simulink model "myMat2"  (R2020b)
settings: Solver=VariableStepAuto  StartTime=0.0  StopTime=200  RelTol=1e-3
libraries: pid_lib x2, simulink x2
settings Model: Creator=jsoudier01  LastModifiedBy=xoxox
settings DataIOCC: ReturnWorkspaceOutputs=off
settings DebuggingCC: ArithmeticOperatorsInVariantConditions=warning
settings SFSimCC: SimUseLocalCustomCode=off  CustomCodeUndefinedFunction=UseInterfaceOnly
settings RTWCC: RTWUseLocalCustomCode=off

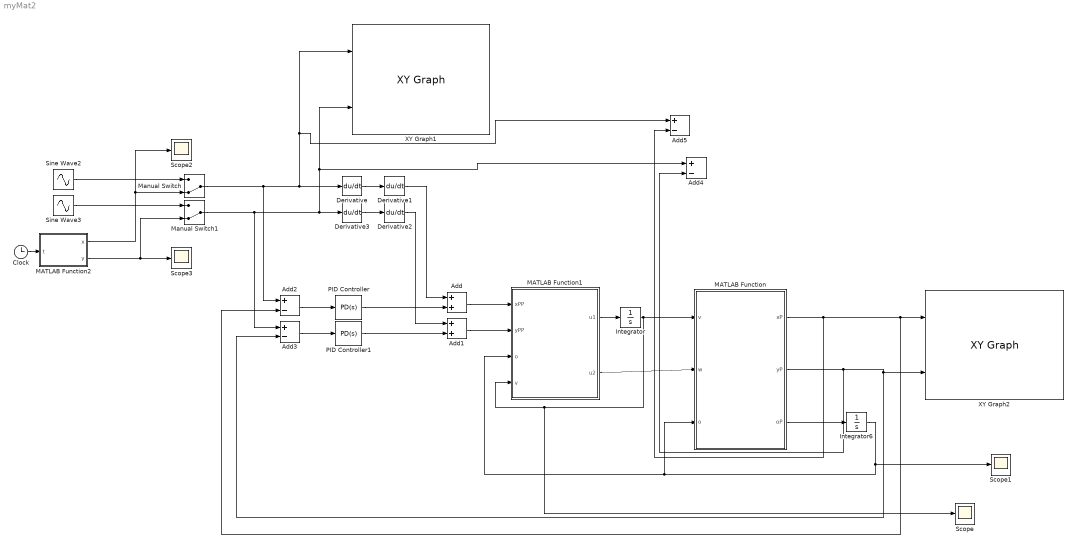
== system myMat2 ==
  Add : Sum
  Add1 : Sum
  Add{2..5} (4 alike) : Sum  Inputs=+-
  Clock : Clock
  Derivative{,1..3} (4 alike) : Derivative
  Integrator : Integrator  InitialCondition=50
  Integrator6 : Integrator  InitialCondition=10
  MATLAB Function : MATLAB Function  TreatAsAtomicUnit=on
  MATLAB Function1 : MATLAB Function  TreatAsAtomicUnit=on
  MATLAB Function2 : MATLAB Function  TreatAsAtomicUnit=on
  Manual Switch : ManualSwitch  CurrentSetting=0
  Manual Switch1 : ManualSwitch  CurrentSetting=0
  PID Controller : pid_lib/PID Controller  Controller=PD  Form=Ideal  TimeDomain=Continuous-time  UseExternalTs=off  SampleTime=-1  IntegratorMethod=Forward Euler  FilterMethod=Forward Euler  ControllerParametersSource=internal  P=1  I=1  D=1  UseFilter=on  N=100  TunerSelectOption=Transfer Function Based (PID Tuner App)  InitialConditionSource=internal  InitialConditionForIntegrator=0  InitialConditionForFilter=0  DifferentiatorICPrevScaledInput=0  ExternalReset=none  TrackingMode=off  Kt=1  LimitOutput=off  SatLimitsSource=internal  UpperSaturationLimit=inf  LowerSaturationLimit=-inf  LinearizeAsGain=on  AntiWindupMode=none  Kb=1  POutMin=[]  POutMax=[]  IOutMin=[]  IOutMax=[]  DOutMin=[]  DOutMax=[]  NOutMin=[]  NOutMax=[]  SumOutMin=[]  SumOutMax=[]  SaturationOutMin=[]  SaturationOutMax=[]  PParamMin=[]  PParamMax=[]  IParamMin=[]  IParamMax=[]  DParamMin=[]  DParamMax=[]  NParamMin=[]  NParamMax=[]  KbParamMin=[]  KbParamMax=[]  KtParamMin=[]  KtParamMax=[]  KbOutMin=[]  KbOutMax=[]  KtOutMin=[]  KtOutMax=[]  IntegratorOutMin=[]  IntegratorOutMax=[]  FilterOutMin=[]  FilterOutMax=[]  SumI1OutMin=[]  SumI1OutMax=[]  SumI2OutMin=[]  SumI2OutMax=[]  SumI3OutMin=[]  SumI3OutMax=[]  SumI4OutMin=[]  SumI4OutMax=[]  SumDOutMin=[]  SumDOutMax=[]  DifferentiatorOutMin=[]  DifferentiatorOutMax=[]  FilterDiffOutCoefMin=[]  FilterDiffOutCoefMax=[]  ReciprocalOutMin=[]  ReciprocalOutMax=[]  SumDenOutMin=[]  SumDenOutMax=[]  SumNumOutMin=[]  SumNumOutMax=[]  DivideOutMin=[]  DivideOutMax=[]  UdiffTsProdOutMin=[]  UdiffTsProdOutMax=[]  NTsProdOutMin=[]  NTsProdOutMax=[]  UintegralTsProdOutMin=[]  UintegralTsProdOutMax=[]  UngainTsProdOutMin=[]  UngainTsProdOutMax=[]  IntegratorContinuousStateAttributes=''  IntegratorStateMustResolveToSignalObject=off  IntegratorRTWStateStorageClass=Auto  FilterContinuousStateAttributes=''  FilterStateMustResolveToSignalObject=off  FilterRTWStateStorageClass=Auto  ParallelPVariant=Passthrough  IdealPVariant=InternalParameters  IVariant=Disabled  DVariant=InternalParameters  IntegratorVariant=Disabled  SatVariant=Disabled  AWVariant=Disabled  PCopyVariant=Disabled  TRVariant=Disabled  FdbkBlocksVariant=Forward  IdealPFdbkVariant=Disabled  SatFdbkVariant=Disabled  DerivativeFilterVariant=ContFilter  NVariant=InternalParameters  NCopyVariant=Disabled  FilterICVariant=InternalICsFilter  IntegratorICVariant=Disabled  ExternalResetVariant=Disabled  TRSumVariant=Passthrough  SumFdbkVariant=Disabled  SumVariant=Sum_PD  TsampFilterVariant=InternalTs  TsampNgainVariant=Passthrough  TsampIntegralVariant=Disabled_SignalSpec  ExternalSaturationOutDataTypeStr=Inherit: Same as second input
  PID Controller1 : pid_lib/PID Controller  Controller=PD  Form=Ideal  TimeDomain=Continuous-time  UseExternalTs=off  SampleTime=-1  IntegratorMethod=Forward Euler  FilterMethod=Forward Euler  ControllerParametersSource=internal  P=1  I=1  D=1  UseFilter=on  N=100  TunerSelectOption=Transfer Function Based (PID Tuner App)  InitialConditionSource=internal  InitialConditionForIntegrator=0  InitialConditionForFilter=0  DifferentiatorICPrevScaledInput=0  ExternalReset=none  TrackingMode=off  Kt=1  LimitOutput=off  SatLimitsSource=internal  UpperSaturationLimit=inf  LowerSaturationLimit=-inf  LinearizeAsGain=on  AntiWindupMode=none  Kb=1  POutMin=[]  POutMax=[]  IOutMin=[]  IOutMax=[]  DOutMin=[]  DOutMax=[]  NOutMin=[]  NOutMax=[]  SumOutMin=[]  SumOutMax=[]  SaturationOutMin=[]  SaturationOutMax=[]  PParamMin=[]  PParamMax=[]  IParamMin=[]  IParamMax=[]  DParamMin=[]  DParamMax=[]  NParamMin=[]  NParamMax=[]  KbParamMin=[]  KbParamMax=[]  KtParamMin=[]  KtParamMax=[]  KbOutMin=[]  KbOutMax=[]  KtOutMin=[]  KtOutMax=[]  IntegratorOutMin=[]  IntegratorOutMax=[]  FilterOutMin=[]  FilterOutMax=[]  SumI1OutMin=[]  SumI1OutMax=[]  SumI2OutMin=[]  SumI2OutMax=[]  SumI3OutMin=[]  SumI3OutMax=[]  SumI4OutMin=[]  SumI4OutMax=[]  SumDOutMin=[]  SumDOutMax=[]  DifferentiatorOutMin=[]  DifferentiatorOutMax=[]  FilterDiffOutCoefMin=[]  FilterDiffOutCoefMax=[]  ReciprocalOutMin=[]  ReciprocalOutMax=[]  SumDenOutMin=[]  SumDenOutMax=[]  SumNumOutMin=[]  SumNumOutMax=[]  DivideOutMin=[]  DivideOutMax=[]  UdiffTsProdOutMin=[]  UdiffTsProdOutMax=[]  NTsProdOutMin=[]  NTsProdOutMax=[]  UintegralTsProdOutMin=[]  UintegralTsProdOutMax=[]  UngainTsProdOutMin=[]  UngainTsProdOutMax=[]  IntegratorContinuousStateAttributes=''  IntegratorStateMustResolveToSignalObject=off  IntegratorRTWStateStorageClass=Auto  FilterContinuousStateAttributes=''  FilterStateMustResolveToSignalObject=off  FilterRTWStateStorageClass=Auto  ParallelPVariant=Passthrough  IdealPVariant=InternalParameters  IVariant=Disabled  DVariant=InternalParameters  IntegratorVariant=Disabled  SatVariant=Disabled  AWVariant=Disabled  PCopyVariant=Disabled  TRVariant=Disabled  FdbkBlocksVariant=Forward  IdealPFdbkVariant=Disabled  SatFdbkVariant=Disabled  DerivativeFilterVariant=ContFilter  NVariant=InternalParameters  NCopyVariant=Disabled  FilterICVariant=InternalICsFilter  IntegratorICVariant=Disabled  ExternalResetVariant=Disabled  TRSumVariant=Passthrough  SumFdbkVariant=Disabled  SumVariant=Sum_PD  TsampFilterVariant=InternalTs  TsampNgainVariant=Passthrough  TsampIntegralVariant=Disabled_SignalSpec  ExternalSaturationOutDataTypeStr=Inherit: Same as second input
  Scope{,1..3} (4 alike) : Scope
  Sine Wave2 : Sin  Frequency=1/10  SampleTime=0
  Sine Wave3 : Sin  Frequency=1/20  SampleTime=0
  XY Graph1 : simulink/Sinks/XY Graph  xmin=-10  xmax=10  ymin=-10  ymax=10  st=-1
  XY Graph2 : simulink/Sinks/XY Graph  xmin=-100  xmax=100  ymin=-100  ymax=100  st=-1
  wires:
  Manual Switch/1 -> Add2/1, Add5/1, XY Graph1/1, Derivative/1
  Derivative/1 -> Derivative1/1
  Manual Switch1/1 -> Add3/1, Add4/1, XY Graph1/2, Derivative3/1
  Derivative3/1 -> Derivative2/1
  MATLAB Function/3(oP) -> Integrator6/1
  Integrator6/1 -> Scope1/1, MATLAB Function1/3(o), MATLAB Function/3(o)
  MATLAB Function1/2(u2) -> MATLAB Function/2(w)
  MATLAB Function1/1(u1) -> Integrator/1
  Integrator/1 -> Scope/1, MATLAB Function1/4(v), MATLAB Function/1(v)
  MATLAB Function/1(xP) -> Add5/2, XY Graph2/1, Add2/2
  MATLAB Function/2(yP) -> Add4/2, XY Graph2/2, Add3/2
  Add/1 -> MATLAB Function1/1(xPP)
  Add1/1 -> MATLAB Function1/2(yPP)
  Derivative1/1 -> Add/1
  Derivative2/1 -> Add1/1
  Add3/1 -> PID Controller1/1
  Add2/1 -> PID Controller/1
  PID Controller/1 -> Add/2
  PID Controller1/1 -> Add1/2
  Sine Wave2/1 -> Manual Switch/1
  Sine Wave3/1 -> Manual Switch1/1
  MATLAB Function2/1(x) -> Scope2/1, Manual Switch/2
  MATLAB Function2/2(y) -> Manual Switch1/2, Scope3/1
  Clock/1 -> MATLAB Function2/1(t)

== matlab function myMat2/MATLAB Function1 ==
  data: u1 output; xPP input; u2 output; yPP input; o input; v input
function [u1,u2] = fcn(xPP,yPP,o,v)
    u = [cos(o) sin(o);-sin(o)/v cos(o)/v]*[xPP;yPP];
    %u1 = (v*xPP*cos(o)+yPP)/(v*cos(o).^2*sin(o));
    %u2 = (yPP*cos(o)-xPP)/(cos(o).^2*sin(o));
    u1 = u(1);
    u2 = u(2);
end

== matlab function myMat2/MATLAB Function ==
  data: v input; xP output; w input; yP output; oP output; o input
function [xP,yP,oP] = fcn(v,w,o)
    xP = v*cos(o);
    yP = v*sin(o);
    oP = w;
end

== matlab function myMat2/MATLAB Function2 ==
  data: t input; x output; y output
function [x,y] = fcn(t)
    TIME_BASE = 12;
    tt = mod(t,TIME_BASE);
    
    if(tt < 4)
        x = 0;
        y = tt;
    else
        if(tt < 5)
            x = (tt-4)^2;
            y = sqrt(tt-4)+4;
            %y = (tt-4)^2+4;
        else
            if(tt < 6)
                x = sqrt(tt-5)+1;
                y = -(tt-5)^2+5;
                %y = -sqrt(tt-5)+5;
            else
                if(tt < 10)
                    x = 2;
                    y = -(tt-6)+4;
                else
                    if(tt < 11)
                        x = -(tt-10)^2+2;
                        y = -sqrt(tt-10);
                    else
                        x = -sqrt(tt-11)+1;
                        y = (tt-11)^2-1;
                    end
                end
            end
        end
    end
end
